simulink model "Proj4_FINAL_INDIVIDUAL"  (R2024b)
settings: Solver=ode15s  StartTime=0.0  StopTime=3600  FixedStep=0.1  MaxStep=1e-2  MinStep=1e-8  RelTol=1e-2  AbsTol=1e-6
values from neighbouring files (symbols this model uses):
  axel_distances = [1.6,1.4]    [Project4_FINAL_INDIVIDUAL_INITIAL.m]
  eta_speed = [0:500:10000]    [Project4_FINAL_INDIVIDUAL_INITIAL.m]
  eta_torque = [0:25:325] * 280/325 * scaleFactor    [Project4_FINAL_INDIVIDUAL_INITIAL.m]
  eta_val = eta_val .* eta_val    [Project4_FINAL_INDIVIDUAL_INITIAL.m]
  g_b = 2.1    [Project4_FINAL_INDIVIDUAL_INITIAL.m]
  gear_ratio = 10    [Project4_FINAL_INDIVIDUAL_INITIAL.m]
  I_w = 1.7    [Project4_FINAL_INDIVIDUAL_INITIAL.m]
  l = 2    [Project4_FINAL_INDIVIDUAL_INITIAL.m]
  lambda_max = 0.1    [Project4_FINAL_INDIVIDUAL_INITIAL.m]
  m = 80    [Project4_FINAL_INDIVIDUAL_INITIAL.m]
  mass_inert = [80,1]    [Project4_FINAL_INDIVIDUAL_INITIAL.m]
  maxtorque = [0, 0, 0, 0, 0, 0,  0,  0,  0,  0,   0,   0,     0 ... (first row only)    [Project4_FINAL_INDIVIDUAL_INITIAL.m]
  mu = 0.8    [Project4_FINAL_INDIVIDUAL_INITIAL.m]
  mu_b = 0.7    [Project4_FINAL_INDIVIDUAL_INITIAL.m]
  N_b_max = 10000    [Project4_FINAL_INDIVIDUAL_INITIAL.m]
  nom_stiff = 50    [Project4_FINAL_INDIVIDUAL_INITIAL.m]
  numParallel = 74    [Project4_FINAL_INDIVIDUAL_INITIAL.m]
  numSeries = 96    [Project4_FINAL_INDIVIDUAL_INITIAL.m]
  OCV = [0, 3.1,3.55,3.68,3.74,3.76,3.78,3.85,3.9,3.95,4.08,4.15]    [Project4_FINAL_INDIVIDUAL_INITIAL.m]
  r_w = 1.4    [Project4_FINAL_INDIVIDUAL_INITIAL.m]
  Rint = 0.1695    [Project4_FINAL_INDIVIDUAL_INITIAL.m]
  rpm = [0,  1000,2000,3000,4000,5000,6000,7000,8000,9000,10000,11000, 12000]    [Project4_FINAL_INDIVIDUAL_INITIAL.m]
  SOC = [0, 0.01,   .1,  .2,  .3,  .4,  .5,  .6, .7,  .8,  .9,   1]    [Project4_FINAL_INDIVIDUAL_INITIAL.m]
  stiffs = [200,180]    [Project4_FINAL_INDIVIDUAL_INITIAL.m]
  v_max = 22    [Project4_FINAL_INDIVIDUAL_INITIAL.m]
  vbus = [250, 350, 500, 600, 700]*scaleFactor    [Project4_FINAL_INDIVIDUAL_INITIAL.m]
  x_center = [x_straightB, x_curveR, x_straightT, x_curveL]    [Project4_FINAL_INDIVIDUAL_INITIAL.m]
  y_center = [y_straightB, y_curveR, y_straightT, y_curveL]    [Project4_FINAL_INDIVIDUAL_INITIAL.m]
libraries: slpidlib x1
settings Model: Creator=davsc  LastModifiedBy=lukep

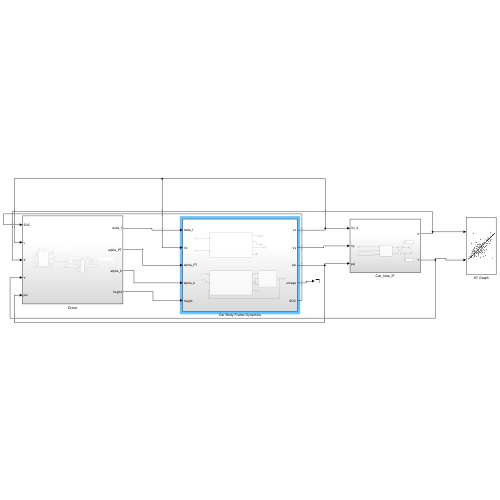
[thumbnail: Simulink's stored preview of the top-level diagram]
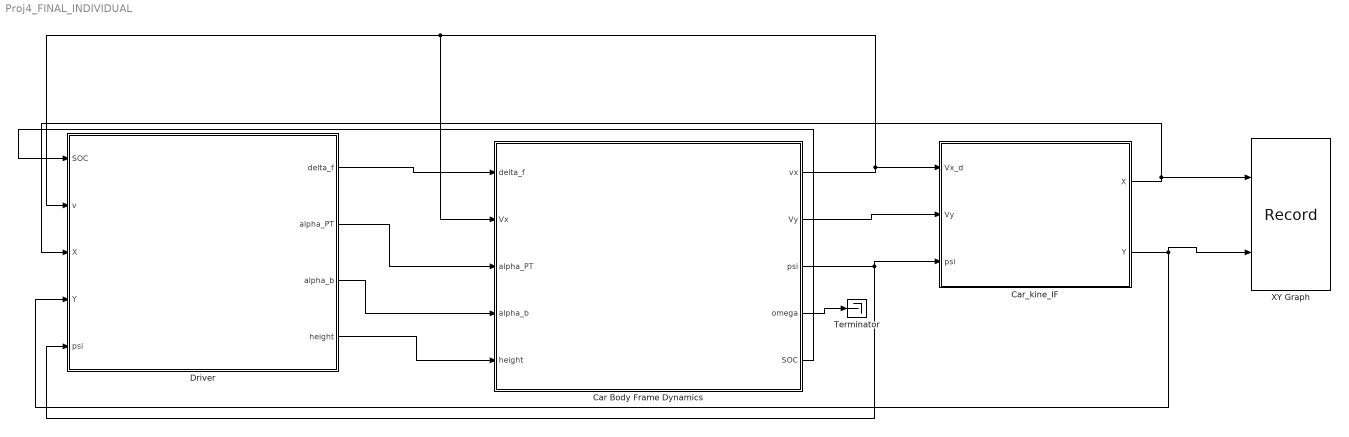
== system Proj4_FINAL_INDIVIDUAL ==
  Car Body Frame Dynamics : Subsystem
  Car_kine_IF : Subsystem
  Driver : Subsystem
  Terminator : Terminator
  XY Graph : Record  FileSettingsInternal="{\"entries\":[{\"content\":{\"excelSettings\":{\"content\":{},\"type\":\"Streamout.ExcelSettings\"}},\"type\":\"Streamout.FileSettingStorage\",\"uuid\":\"\"}],\"packageUris\":[\"http:\\/\\/schema.mathworks.com\\/mf0\\/streamout_blocks\\/R2020a\"],\"version\":\"1.0\"}"  Layout=[1 1]  SignalsInternal="{\"entries\":[{\"content\":{\"signals\":[{\"content\":{\"blockPath\":[],\"dimensions\":[1],\"domain\":\"\",\"lineColor\":\"#edb120\",\"lineWidth\":2,\"port\":1,\"sid\":[\"\"],\"signalID\":1,\"signalName\":\"Car_kine_IF:1\"},\"type\":\"RecordBlkView.Signal\",\"uuid\":\"\"},{\"content\":{\"blockPath\":[],\"dimensions\":[1],\"domain\":\"\",\"lineColor\":\"#7e2f8e\",\"lineWidth\":2,\"port\":2,\"sid\":[\"\"],\"signalID\":2,\"signalName\":\"Car_kine_IF:2\"},\"type\":\"RecordBlkView.Signal\",\"uuid\":\"\"},{\"content\":{\"blockPath\":[],\"dimensions\":[1],\"domain\":\"\",\"lineColor\":\"#77ac30\",\"lineWidth\":2,\"port\":1,\"sid\":[\"\"],\"signalID\":3,\"signalName\":\"MATLAB Function\"},\"type\":\"RecordBlkView.Signal\",\"uuid\":\"\"},{\"content\":{\"blockPath\":[],\"dimensions\":[1],\"domain\":\"\",\"lineColor\":\"#4dbeee\",\"lineWidth\":2,\"port\":1,\"sid\":[\"\"],\"signalID\":4,\"signalName\":\"Integrator\"},\"type\":\"RecordBlkView.Signal\",\"uuid\":\"\"},{\"content\":{\"blockPath\":[],\"dimensions\":[1],\"domain\":\"\",\"lineColor\":\"#a2142f\",\"lineWidth\":2,\"port\":1,\"sid\":[\"\"],\"signalID\":5,\"signalName\":\"Electric Motor Drive:5\"},\"type\":\"RecordBlkView.Signal\",\"uuid\":\"\"},{\"content\":{\"blockPath\":[],\"dimensions\":[1],\"domain\":\"\",\"lineColor\":\"#139fff\",\"lineWidth\":2,\"port\":1,\"sid\":[\"\"],\"signalID\":6,\"signalName\":\"1-D Lookup\\nTable\"},\"type\":\"RecordBlkView.Signal\",\"uuid\":\"\"},{\"content\":{\"blockPath\":[],\"dimensions\":[1],\"domain\":\"\",\"lineColor\":\"#ff6929\",\"lineWidth\":2,\"port\":1,\"sid\":[\"\"],\"signalID\":7,\"signalName\":\"gainn\"},\"type\":\"RecordBlkView.Signal\",\"uuid\":\"\"},{\"content\":{\"blockPath\":[],\"dimensions\":[1],\"domain\":\"\",\"lineColor\":\"#b746ff\",\"lineWidth\":2,\"port\":1,\"sid\":[\"\"],\"signalID\":8,\"signalName\":\"Integrator1\"},\"type\":\"RecordBlkView.Signal\",\"uuid\":\"\"},{\"content\":{\"blockPath\":[],\"dimensions\":[1],\"domain\":\"\",\"lineColor\":\"#64d413\",\"lineWidth\":2,\"port\":1,\"sid\":[\"\"],\"signalID\":9,\"signalName\":\"Motor Efficiency Table\"},\"type\":\"RecordBlkView.Signal\",\"uuid\":\"\"},{\"content\":{\"blockPath\":[],\"dimensions\":[1],\"domain\":\"\",\"lineColor\":\"#ff13a6\",\"lineWidth\":2,\"port\":1,\"sid\":[\"\"],\"signalID\":10,\"signalName\":\"Product1\"},\"type\":\"RecordBlkView.Signal\",\"uuid\":\"\"},{\"content\":{\"blockPath\":[],\"dimensions\":[1],\"domain\":\"\",\"lineColor\":\"#fe330a\",\"lineWidth\":2,\"port\":1,\"sid\":[\"\"],\"signalID\":11,\"signalName\":\"Integrator\"},\"type\":\"RecordBlkView.Signal\",\"uuid\":\"\"},{\"content\":{\"blockPath\":[],\"dimensions\":[1],\"domain\":\"\",\"lineColor\":\"#22b573\",\"lineWidth\":2,\"port\":1,\"sid\":[\"\"],\"signalID\":12,\"signalName\":\"MATLAB Function1:1\"},\"type\":\"RecordBlkView.Signal\",\"uuid\":\"\"},{\"content\":{\"blockPath\":[],\"dimensions\":[1],\"domain\":\"\",\"lineColor\":\"#0072bd\",\"lineWidth\":2,\"port\":1,\"sid\":[\"\"],\"signalID\":13,\"signalName\":\"MATLAB Function1:2\"},\"type\":\"RecordBlkView.Signal\",\"uuid\":\"\"},{\"content\":{\"blockPath\":[],\"dimensions\":[1],\"domain\":\"\",\"lineColor\":\"#d95319\",\"lineWidth\":2,\"port\":1,\"sid\":[\"\"],\"signalID\":14,\"signalName\":\"MATLAB Function2:1\"},\"type\":\"RecordBlkView.Signal\",\"uuid\":\"\"},{\"content\":{\"blockPath\":[],\"dimensions\":[1],\"domain\":\"\",\"lineColor\":\"#edb120\",\"lineWidth\":2,\"port\":1,\"sid\":[\"\"],\"signalID\":15,\"signalName\":\"MATLAB Function2:2\"},\"type\":\"RecordBlkView.Signal\",\"uuid\":\"\"},{\"content\":{\"blockPath\":[],\"dimensions\":[1],\"domain\":\"\",\"lineColor\":\"#7e2f8e\",\"lineWidth\":2,\"port\":1,\"sid\":[\"\"],\"signalID\":16,\"signalName\":\"Integrator2\"},\"type\":\"RecordBlkView.Signal\",\"uuid\":\"\"},{\"content\":{\"blockPath\":[],\"dimensions\":[1],\"domain\":\"\",\"lineColor\":\"#77ac30\",\"lineWidth\":2,\"port\":1,\"sid\":[\"\"],\"signalID\":17,\"signalName\":\"Integrator1\"},\"type\":\"RecordBlkView.Signal\",\"uuid\":\"\"},{\"content\":{\"blockPath\":[],\"dimensions\":[1],\"domain\":\"\",\"lineColor\":\"#4dbeee\",\"lineWidth\":2,\"port\":1,\"sid\":[\"\"],\"signalID\":18,\"signalName\":\"Integrator4\"},\"type\":\"RecordBlkView.Signal\",\"uuid\":\"\"},{\"content\":{\"blockPath\":[],\"dimensions\":[1],\"domain\":\"\",\"lineColor\":\"#a2142f\",\"lineWidth\":2,\"port\":1,\"sid\":[\"\"],\"signalID\":19,\"signalName\":\"Integrator\"},\"type\":\"RecordBlkView.Signal\",\"uuid\":\"\"},{\"content\":{\"blockPath\":[],\"dimensions\":[1],\"domain\":\"\",\"lineColor\":\"#139fff\",\"lineWidth\":2,\"port\":1,\"sid\":[\"\"],\"signalID\":20,\"signalName\":\"Integrator1\"},\"type\":\"RecordBlkView.Signal\",\"uuid\":\"\"},{\"content\":{\"blockPath\":[],\"dimensions\":[1],\"domain\":\"\",\"lineColor\":\"#ff6929\",\"lineWidth\":2,\"port\":1,\"sid\":[\"\"],\"signalID\":21,\"signalName\":\"MATLAB Function:1\"},\"type\":\"RecordBlkView.Signal\",\"uuid\":\"\"},{\"content\":{\"blockPath\":[],\"dimensions\":[1],\"domain\":\"\",\"lineColor\":\"#b746ff\",\"lineWidth\":2,\"port\":1,\"sid\":[\"\"],\"signalID\":22,\"signalName\":\"MATLAB Function:2\"},\"type\":\"RecordBlkView.Signal\",\"uuid\":\"\"}]},\"type\":\"RecordBlkView.InputSignals\",\"uuid\":\"\"}],\"packageUris\":[\"http:\\/\\/schema.mathworks.com\\/mf0\\/streamout_blocks\\/R2020a\"],\"version\":\"1.0\"}"  VisualizationBindings="{\"xyplotplugin\":{\"info\":[{\"series\":[],\"subplotID\":1}]}}"  CompatibilityTag=XY
  wires:
  Driver/2(alpha_PT) -> Car Body Frame Dynamics/3(alpha_PT)
  Driver/3(alpha_b) -> Car Body Frame Dynamics/4(alpha_b)
  Car Body Frame Dynamics/4(omega) -> Terminator/1
  Car Body Frame Dynamics/5(SOC) -> Driver/1(SOC)
  Car Body Frame Dynamics/1(vx) -> Car Body Frame Dynamics/2(Vx), Driver/2(v), Car_kine_IF/1(Vx_d)
  Car Body Frame Dynamics/2(Vy) -> Car_kine_IF/2(Vy)
  Car Body Frame Dynamics/3(psi) -> Car_kine_IF/3(psi), Driver/5(psi)
  Car_kine_IF/1(X) -> Driver/3(X), XY Graph/1
  Car_kine_IF/2(Y) -> XY Graph/2, Driver/4(Y)
  Driver/1(delta_f) -> Car Body Frame Dynamics/1(delta_f)
  Driver/4(height) -> Car Body Frame Dynamics/5(height)

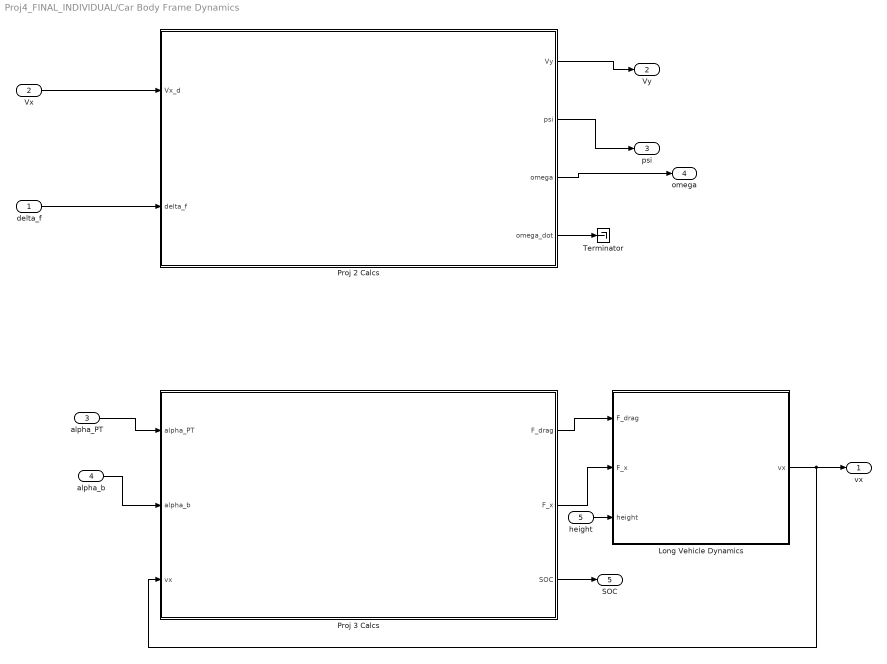
== system Proj4_FINAL_INDIVIDUAL/Car Body Frame Dynamics ==
  delta_f : Inport
  Vx : Inport  Port=2
  alpha_PT : Inport  Port=3
  alpha_b : Inport  Port=4
  height : Inport  Port=5
  Long Vehicle Dynamics : Subsystem
  Proj 2 Calcs : Subsystem
  Proj 3 Calcs : Subsystem
  Terminator : Terminator
  vx : Outport
  Vy : Outport  Port=2
  psi : Outport  Port=3
  omega : Outport  Port=4
  SOC : Outport  Port=5
  wires:
  alpha_PT/1 -> Proj 3 Calcs/1(alpha_PT)
  alpha_b/1 -> Proj 3 Calcs/2(alpha_b)
  Vx/1 -> Proj 2 Calcs/1(Vx_d)
  delta_f/1 -> Proj 2 Calcs/2(delta_f)
  Proj 3 Calcs/2(F_x) -> Long Vehicle Dynamics/2(F_x)
  Proj 3 Calcs/1(F_drag) -> Long Vehicle Dynamics/1(F_drag)
  Proj 3 Calcs/3(SOC) -> SOC/1
  Proj 2 Calcs/1(Vy) -> Vy/1
  Proj 2 Calcs/2(psi) -> psi/1
  Proj 2 Calcs/3(omega) -> omega/1
  Long Vehicle Dynamics/1(vx) -> Proj 3 Calcs/3(vx), vx/1
  Proj 2 Calcs/4(omega_dot) -> Terminator/1
  height/1 -> Long Vehicle Dynamics/3(height)

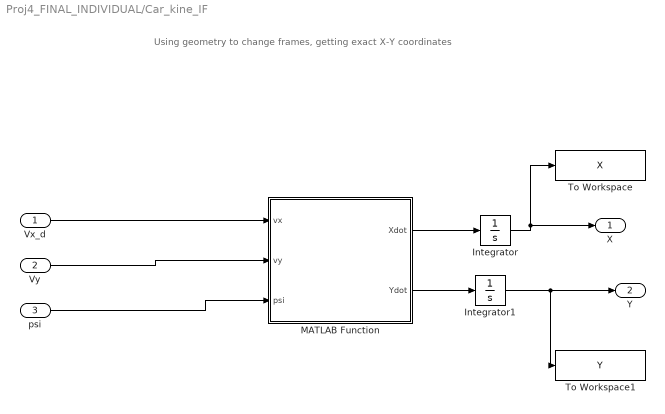
== system Proj4_FINAL_INDIVIDUAL/Car_kine_IF ==
  note: Using geometry to change frames, getting exact X-Y coordinates
  Vx_d : Inport
  Vy : Inport  Port=2
  psi : Inport  Port=3
  Integrator : Integrator
  Integrator1 : Integrator
  MATLAB Function : MATLAB Function  TreatAsAtomicUnit=on
  To Workspace : ToWorkspace  VariableName=X  SaveFormat=Timeseries  SampleTime=0.5
  To Workspace1 : ToWorkspace  VariableName=Y  SaveFormat=Timeseries  SampleTime=0.5
  X : Outport
  Y : Outport  Port=2
  wires:
  Vx_d/1 -> MATLAB Function/1(vx)
  psi/1 -> MATLAB Function/3(psi)
  Vy/1 -> MATLAB Function/2(vy)
  MATLAB Function/1(Xdot) -> Integrator/1
  MATLAB Function/2(Ydot) -> Integrator1/1
  Integrator1/1 -> To Workspace1/1, Y/1
  Integrator/1 -> To Workspace/1, X/1

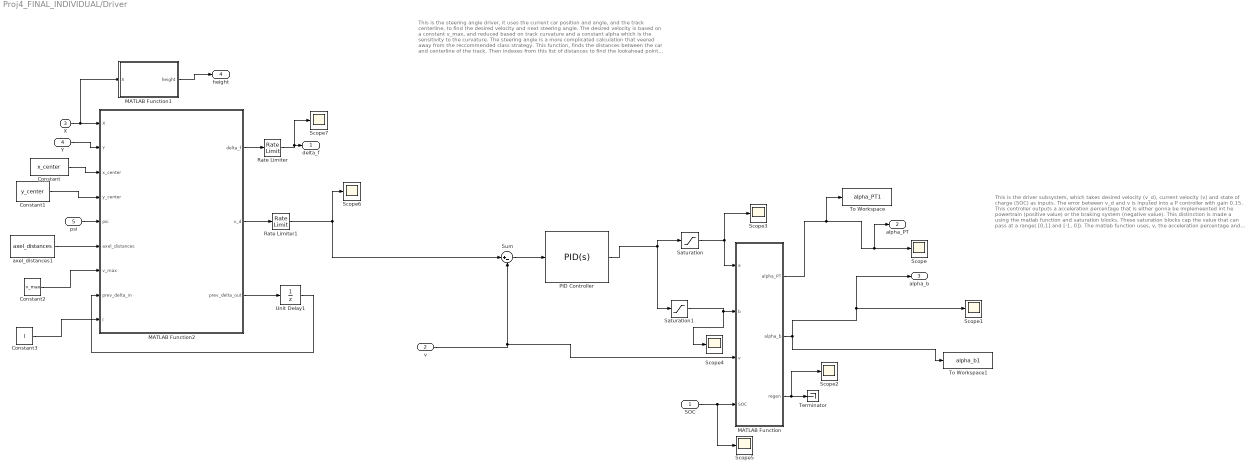
== system Proj4_FINAL_INDIVIDUAL/Driver ==
  note: This is the steering angle driver, it uses the current car position and angle, and the track centerline, to find the desired velocity and next steering angle. The desired velocity is based on a constant v_max, and reduced based on track curvature and a constant alpha which is the sensitivity to the curvature. The steering angle is a more complicated calculation that veered away from the reccommended class strategy. This function, finds the distances between the car and centerline of the track. Then indexes from this list of distances to find the lookahead point on the centerline (distance l). Then steering angle is simply calculated once lookahead point is found (psi_d to error to dleta_f). Where steering angle and desired speed is capped to keep the car on the track as much as possible
  note: This is the driver subsystem, which takes desired velocity (v_d), current velocity (v) and state of charge (SOC) as inputs. The error between v_d and v is inputed into a P controller with gain 0.15. This controller outputs a acceleration percentage that is either gonna be implemeented int he powertrain (positive value) or the braking system (negative value). This distinction is made a using the matlab function and saturation blocks. These saturation blocks cap the value that can pass at a range( [0,1] and [-1, 0]). The matlab function uses, v, the acceleration percentage and SOC, to output the brake or powertrain accerlation and a regeneration factor. The logic of this function accelerates the vehicle based on current speed and current SOC.
  SOC : Inport
  v : Inport  Port=2
  X : Inport  Port=3
  Y : Inport  Port=4
  psi : Inport  Port=5
  Constant : Constant  Value=x_center
  Constant1 : Constant  Value=y_center
  Constant2 : Constant  Value=v_max
  Constant3 : Constant  Value=l
  MATLAB Function : MATLAB Function  TreatAsAtomicUnit=on
  MATLAB Function1 : MATLAB Function  TreatAsAtomicUnit=on
  MATLAB Function2 : MATLAB Function  TreatAsAtomicUnit=on
  PID Controller : slpidlib/PID Controller  Controller=PID  Form=Parallel  TimeDomain=Continuous-time  UseExternalTs=off  SampleTime=-1  IntegratorMethod=Forward Euler  FilterMethod=Forward Euler  ControllerParametersSource=internal  P=0.5  I=0  UseKiTs=off  D=0  UseExternalDerivativeSource=off  N=100  UseFilter=on  TunerSelectOption=Transfer Function Based (PID Tuner App)  InitialConditionSource=internal  InitialConditionForIntegrator=0  InitialConditionForFilter=0  DifferentiatorICPrevScaledInput=0  ExternalReset=none  TrackingMode=off  Kt=1  LimitOutput=off  SatLimitsSource=internal  UpperSaturationLimit=inf  LowerSaturationLimit=-inf  LinearizeAsGain=on  AntiWindupMode=none  Kb=1  LimitIntegrator=off  UpperIntegratorSaturationLimit=inf  LowerIntegratorSaturationLimit=-inf  POutMin=[]  POutMax=[]  IOutMin=[]  IOutMax=[]  DOutMin=[]  DOutMax=[]  NOutMin=[]  NOutMax=[]  SumOutMin=[]  SumOutMax=[]  SaturationOutMin=[]  SaturationOutMax=[]  PParamMin=[]  PParamMax=[]  IParamMin=[]  IParamMax=[]  DParamMin=[]  DParamMax=[]  NParamMin=[]  NParamMax=[]  KbParamMin=[]  KbParamMax=[]  KtParamMin=[]  KtParamMax=[]  KbOutMin=[]  KbOutMax=[]  KtOutMin=[]  KtOutMax=[]  IntegratorOutMin=[]  IntegratorOutMax=[]  FilterOutMin=[]  FilterOutMax=[]  SumI1OutMin=[]  SumI1OutMax=[]  SumI2OutMin=[]  SumI2OutMax=[]  SumI3OutMin=[]  SumI3OutMax=[]  SumI4OutMin=[]  SumI4OutMax=[]  SumDOutMin=[]  SumDOutMax=[]  DifferentiatorOutMin=[]  DifferentiatorOutMax=[]  FilterDiffOutCoefMin=[]  FilterDiffOutCoefMax=[]  ReciprocalOutMin=[]  ReciprocalOutMax=[]  SumDenOutMin=[]  SumDenOutMax=[]  SumNumOutMin=[]  SumNumOutMax=[]  DivideOutMin=[]  DivideOutMax=[]  UdiffTsProdOutMin=[]  UdiffTsProdOutMax=[]  NTsProdOutMin=[]  NTsProdOutMax=[]  UintegralTsProdOutMin=[]  UintegralTsProdOutMax=[]  UngainTsProdOutMin=[]  UngainTsProdOutMax=[]  ClampingZeroOutDataTypeStr=Inherit: Inherit via back propagation  ClampingZeroOutMin=[]  ClampingZeroOutMax=[]  FilterDenConstantOutDataTypeStr=Inherit: Inherit via back propagation  FilterDenConstantOutMin=[]  FilterDenConstantOutMax=[]  PCopyOutDataTypeStr=Inherit: Inherit via back propagation  PCopyOutMin=[]  PCopyOutMax=[]  NCopyOutDataTypeStr=Inherit: Inherit via back propagation  NCopyOutMin=[]  NCopyOutMax=[]  IntegratorContinuousStateAttributes=''  IntegratorStateMustResolveToSignalObject=off  IntegratorRTWStateStorageClass=Auto  FilterContinuousStateAttributes=''  FilterStateMustResolveToSignalObject=off  FilterRTWStateStorageClass=Auto  ParallelPVariant=InternalParameters  IdealPVariant=Disabled  IVariant=InternalParameters  DVariant=InternalParameters  IntegratorVariant=Continuous  SatVariant=Disabled  AWVariant=Passthrough  PCopyVariant=Disabled  TRVariant=Disabled  FdbkBlocksVariant=Forward  IdealPFdbkVariant=Disabled  SatFdbkVariant=Disabled  DerivativeFilterVariant=ContFilter  NVariant=InternalParameters  NCopyVariant=Disabled  FilterICVariant=InternalICsFilter  IntegratorICVariant=InternalICs  ExternalResetVariant=Disabled  TRSumVariant=Passthrough  SumFdbkVariant=Disabled  SumVariant=Sum_PID  TsampFilterVariant=InternalTs  TsampNgainVariant=Passthrough  TsampIntegralVariant=Disabled_SignalSpec  ExternalSaturationOutDataTypeStr=Inherit: Same as second input  DerivativeSourceVariant=ErrorSignal  PreIntVariant=InternalPreInt
  Rate Limiter : RateLimiter  SampleTimeMode=inherited
  Rate Limiter1 : RateLimiter  SampleTimeMode=inherited
  Saturation : Saturate  UpperLimit=1  LowerLimit=0
  Saturation1 : Saturate  UpperLimit=0  LowerLimit=-1
  Scope{,1..7} (8 alike) : Scope
  Sum : Sum  Inputs=|+-
  Terminator : Terminator
  To Workspace : ToWorkspace  VariableName=alpha_PT1  SaveFormat=Timeseries  SampleTime=-1
  To Workspace1 : ToWorkspace  VariableName=alpha_b1  SaveFormat=Timeseries  SampleTime=-1
  Unit Delay1 : UnitDelay  SampleTime=-1  HasFrameUpgradeWarning=on
  axel_distances1 : Constant  Value=axel_distances
  delta_f : Outport
  alpha_PT : Outport  Port=2
  alpha_b : Outport  Port=3
  height : Outport  Port=4
  wires:
  Sum/1 -> PID Controller/1
  PID Controller/1 -> Saturation/1, Saturation1/1
  MATLAB Function2/2(v_d) -> Rate Limiter1/1
  MATLAB Function/2(alpha_b) -> alpha_b/1, Scope1/1, To Workspace1/1
  MATLAB Function/3(regen) -> Scope2/1, Terminator/1
  Saturation1/1 -> Scope4/1, MATLAB Function/2(b)
  SOC/1 -> Scope5/1, MATLAB Function/4(SOC)
  Saturation/1 -> MATLAB Function/1(a), Scope3/1
  v/1 -> MATLAB Function/3(v), Sum/2
  MATLAB Function/1(alpha_PT) -> To Workspace/1, Scope/1, alpha_PT/1
  axel_distances1/1 -> MATLAB Function2/6(axel_distances)
  MATLAB Function2/3(prev_delta_out) -> Unit Delay1/1
  Constant3/1 -> MATLAB Function2/9(l)
  Constant2/1 -> MATLAB Function2/7(v_max)
  Constant1/1 -> MATLAB Function2/4(y_center)
  X/1 -> MATLAB Function1/1(X), MATLAB Function2/1(X)
  Y/1 -> MATLAB Function2/2(Y)
  Constant/1 -> MATLAB Function2/3(x_center)
  psi/1 -> MATLAB Function2/5(psi)
  Unit Delay1/1 -> MATLAB Function2/8(prev_delta_in)
  MATLAB Function2/1(delta_f) -> Rate Limiter/1
  Rate Limiter/1 -> Scope7/1, delta_f/1
  Rate Limiter1/1 -> Scope6/1, Sum/1
  MATLAB Function1/1(height) -> height/1

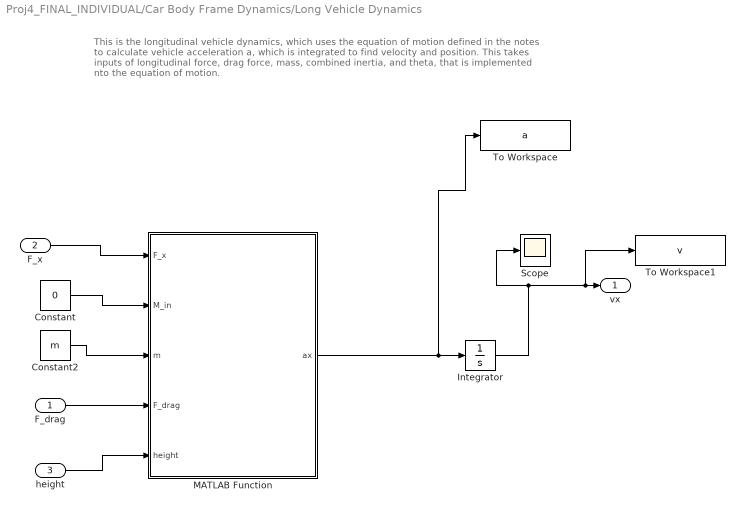
== system Proj4_FINAL_INDIVIDUAL/Car Body Frame Dynamics/Long Vehicle Dynamics ==
  note: This is the longitudinal vehicle dynamics, which uses the equation of motion defined in the notes to calculate vehicle acceleration a, which is integrated to find velocity and position. This takes inputs of longitudinal force, drag force, mass, combined inertia, and theta, that is implemented nto the equation of motion.
  F_drag : Inport
  F_x : Inport  Port=2
  height : Inport  Port=3
  Constant : Constant  Value=0
  Constant2 : Constant  Value=m
  Integrator : Integrator  InitialCondition=0.1
  MATLAB Function : MATLAB Function  TreatAsAtomicUnit=on
  Scope : Scope
  To Workspace : ToWorkspace  VariableName=a  SaveFormat=Timeseries  SampleTime=-1
  To Workspace1 : ToWorkspace  VariableName=v  SaveFormat=Timeseries  SampleTime=-1
  vx : Outport
  wires:
  F_drag/1 -> MATLAB Function/4(F_drag)
  F_x/1 -> MATLAB Function/1(F_x)
  Constant/1 -> MATLAB Function/2(M_in)
  Constant2/1 -> MATLAB Function/3(m)
  MATLAB Function/1(ax) -> To Workspace/1, Integrator/1
  Integrator/1 -> Scope/1, To Workspace1/1, vx/1
  height/1 -> MATLAB Function/5(height)

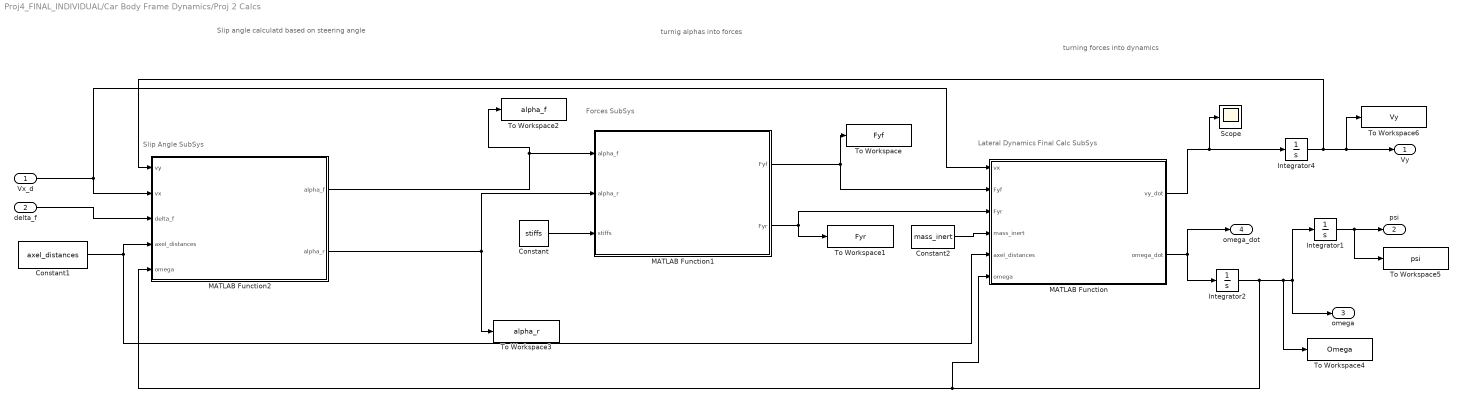
== system Proj4_FINAL_INDIVIDUAL/Car Body Frame Dynamics/Proj 2 Calcs ==
  note: turning forces into dynamics
  note: turnig alphas into forces
  note: Slip angle calculatd based on steering angle
  note: Forces SubSys
  note: Slip Angle SubSys
  note: Lateral Dynamics Final Calc SubSys
  Vx_d : Inport
  delta_f : Inport  Port=2
  Constant : Constant  Value=stiffs
  Constant1 : Constant  Value=axel_distances
  Constant2 : Constant  Value=mass_inert
  Integrator1 : Integrator
  Integrator2 : Integrator
  Integrator4 : Integrator
  MATLAB Function : MATLAB Function  TreatAsAtomicUnit=on
  MATLAB Function1 : MATLAB Function  TreatAsAtomicUnit=on
  MATLAB Function2 : MATLAB Function  TreatAsAtomicUnit=on
  Scope : Scope
  To Workspace : ToWorkspace  VariableName=Fyf  SaveFormat=Timeseries  SampleTime=-1
  To Workspace1 : ToWorkspace  VariableName=Fyr  SaveFormat=Timeseries  SampleTime=-1
  To Workspace2 : ToWorkspace  VariableName=alpha_f  SaveFormat=Timeseries  SampleTime=-1
  To Workspace3 : ToWorkspace  VariableName=alpha_r  SaveFormat=Timeseries  SampleTime=-1
  To Workspace4 : ToWorkspace  VariableName=Omega  SaveFormat=Timeseries  SampleTime=-1
  To Workspace5 : ToWorkspace  VariableName=psi  SaveFormat=Timeseries  SampleTime=-1
  To Workspace6 : ToWorkspace  VariableName=Vy  SaveFormat=Timeseries  SampleTime=-1
  Vy : Outport
  psi : Outport  Port=2
  omega : Outport  Port=3
  omega_dot : Outport  Port=4
  wires:
  Vx_d/1 -> MATLAB Function/1(vx), MATLAB Function2/2(vx)
  Integrator4/1 -> MATLAB Function2/1(vy), To Workspace6/1, Vy/1
  MATLAB Function/1(vy_dot) -> Scope/1, Integrator4/1
  Constant1/1 -> MATLAB Function/5(axel_distances), MATLAB Function2/4(axel_distances)
  Integrator1/1 -> To Workspace5/1, psi/1
  MATLAB Function2/2(alpha_r) -> MATLAB Function1/2(alpha_r), To Workspace3/1
  MATLAB Function1/1(Fyf) -> MATLAB Function/2(Fyf), To Workspace/1
  delta_f/1 -> MATLAB Function2/3(delta_f)
  MATLAB Function/2(omega_dot) -> omega_dot/1, Integrator2/1
  Integrator2/1 -> MATLAB Function2/5(omega), MATLAB Function/6(omega), To Workspace4/1, Integrator1/1, omega/1
  Constant2/1 -> MATLAB Function/4(mass_inert)
  MATLAB Function2/1(alpha_f) -> To Workspace2/1, MATLAB Function1/1(alpha_f)
  Constant/1 -> MATLAB Function1/3(stiffs)
  MATLAB Function1/2(Fyr) -> MATLAB Function/3(Fyr), To Workspace1/1

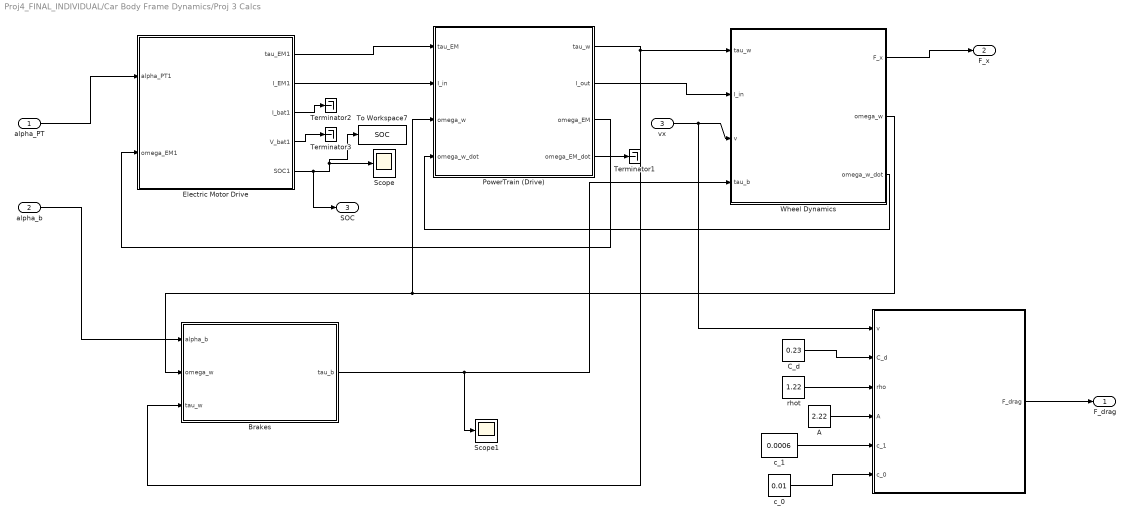
== system Proj4_FINAL_INDIVIDUAL/Car Body Frame Dynamics/Proj 3 Calcs ==
  alpha_PT : Inport
  alpha_b : Inport  Port=2
  vx : Inport  Port=3
  " " : Subsystem
  A : Constant  Value=2.22
  Brakes : Subsystem
  C_d : Constant  Value=0.23
  Electric Motor Drive : Subsystem
  PowerTrain (Drive) : Subsystem
  Scope : Scope
  Scope1 : Scope
  Terminator1 : Terminator
  Terminator2 : Terminator
  Terminator3 : Terminator
  To Workspace7 : ToWorkspace  VariableName=SOC  SaveFormat=Timeseries  SampleTime=-1
  Wheel Dynamics : Subsystem
  c_0 : Constant  Value=0.01
  c_1 : Constant  Value=0.0006
  rhot : Constant  Value=1.22
  F_drag : Outport
  F_x : Outport  Port=2
  SOC : Outport  Port=3
  wires:
  Electric Motor Drive/5(SOC1) -> SOC/1, To Workspace7/1, Scope/1
  A/1 -> " "/4(A)
  Electric Motor Drive/4(V_bat1) -> Terminator3/1
  c_0/1 -> " "/6(c_0)
  rhot/1 -> " "/3(rho)
  Wheel Dynamics/2(omega_w) -> PowerTrain (Drive)/3(omega_w), Brakes/2(omega_w)
  PowerTrain (Drive)/2(I_out) -> Wheel Dynamics/2(I_in)
  Brakes/1(tau_b) -> Scope1/1, Wheel Dynamics/4(tau_b)
  PowerTrain (Drive)/4(omega_EM_dot) -> Terminator1/1
  PowerTrain (Drive)/3(omega_EM) -> Electric Motor Drive/2(omega_EM1)
  Wheel Dynamics/3(omega_w_dot) -> PowerTrain (Drive)/4(omega_w_dot)
  alpha_b/1 -> Brakes/1(alpha_b)
  c_1/1 -> " "/5(c_1)
  PowerTrain (Drive)/1(tau_w) -> Brakes/3(tau_w), Wheel Dynamics/1(tau_w)
  C_d/1 -> " "/2(C_d)
  alpha_PT/1 -> Electric Motor Drive/1(alpha_PT1)
  Electric Motor Drive/1(tau_EM1) -> PowerTrain (Drive)/1(tau_EM)
  Electric Motor Drive/2(I_EM1) -> PowerTrain (Drive)/2(I_in)
  " "/1(F_drag) -> F_drag/1
  Wheel Dynamics/1(F_x) -> F_x/1
  vx/1 -> Wheel Dynamics/3(v), " "/1(v)
  Electric Motor Drive/3(I_bat1) -> Terminator2/1

== system Proj4_FINAL_INDIVIDUAL/Car Body Frame Dynamics/Proj 3 Calcs/  ==
  note: Drag force Subsystem, using constants and current velocity. Implemented in matlab function using given formula in notes.
  v : Inport
  C_d : Inport  Port=2
  rho : Inport  Port=3
  A : Inport  Port=4
  c_1 : Inport  Port=5
  c_0 : Inport  Port=6
  Drag_force : MATLAB Function  TreatAsAtomicUnit=on
  F_drag : Outport
  wires:
  Drag_force/1(F_drag) -> F_drag/1
  C_d/1 -> Drag_force/4(C_d)
  A/1 -> Drag_force/3(A)
  rho/1 -> Drag_force/2(rho)
  v/1 -> Drag_force/1(v)
  c_0/1 -> Drag_force/6(c_0)
  c_1/1 -> Drag_force/5(c_1)

== system Proj4_FINAL_INDIVIDUAL/Car Body Frame Dynamics/Proj 3 Calcs/Brakes ==
  note: This is the brakes subsystem. This takes brake percentage, wheel angular speed (omega_w), and defined constants: max brake force (N_b_max), brake friction (mu_b), and geometric design factor (g_b), and outputs brake torque (tau_b). This is implemented using a given formula in the notes.
  alpha_b : Inport
  omega_w : Inport  Port=2
  tau_w : Inport  Port=3
  Constant : Constant  Value=N_b_max
  Constant1 : Constant  Value=g_b
  Constant2 : Constant  Value=mu_b
  MATLAB Function : MATLAB Function  TreatAsAtomicUnit=on
  tau_b : Outport
  wires:
  Constant2/1 -> MATLAB Function/4(mu_b)
  Constant1/1 -> MATLAB Function/3(g_b)
  Constant/1 -> MATLAB Function/2(N_b_max)
  alpha_b/1 -> MATLAB Function/1(alpha_b)
  omega_w/1 -> MATLAB Function/5(omega_w)
  MATLAB Function/1(tau_b) -> tau_b/1
  tau_w/1 -> MATLAB Function/6(tau_w)

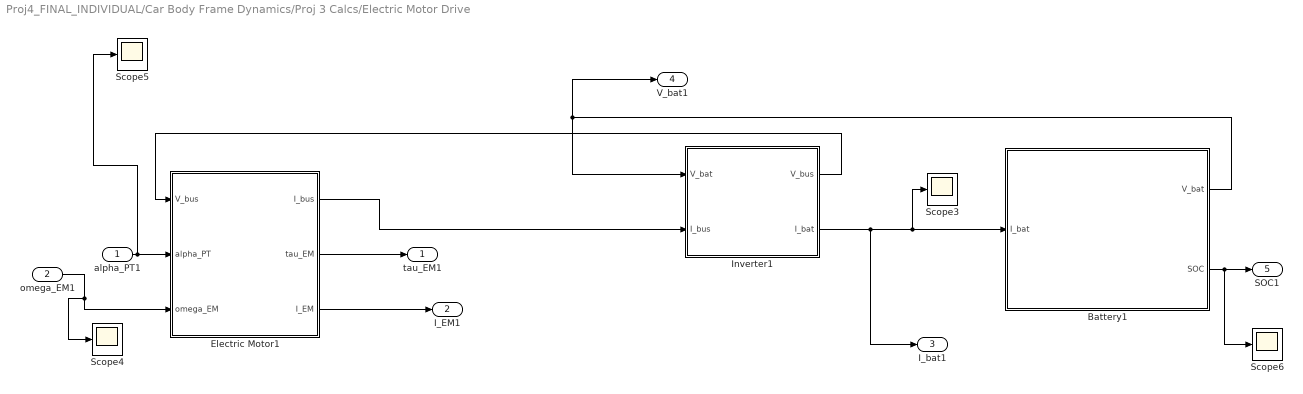
== system Proj4_FINAL_INDIVIDUAL/Car Body Frame Dynamics/Proj 3 Calcs/Electric Motor Drive ==
  alpha_PT1 : Inport
  omega_EM1 : Inport  Port=2
  Battery1 : Subsystem
  Electric Motor1 : Subsystem
  Inverter1 : Subsystem
  Scope{3..6} (4 alike) : Scope
  tau_EM1 : Outport
  I_EM1 : Outport  Port=2
  I_bat1 : Outport  Port=3
  V_bat1 : Outport  Port=4
  SOC1 : Outport  Port=5
  wires:
  Battery1/2(SOC) -> Scope6/1, SOC1/1
  alpha_PT1/1 -> Scope5/1, Electric Motor1/2(alpha_PT)
  Inverter1/1(V_bus) -> Electric Motor1/1(V_bus)
  Battery1/1(V_bat) -> Inverter1/1(V_bat), V_bat1/1
  Electric Motor1/1(I_bus) -> Inverter1/2(I_bus)
  Inverter1/2(I_bat) -> Scope3/1, Battery1/1(I_bat), I_bat1/1
  omega_EM1/1 -> Scope4/1, Electric Motor1/3(omega_EM)
  Electric Motor1/3(I_EM) -> I_EM1/1
  Electric Motor1/2(tau_EM) -> tau_EM1/1

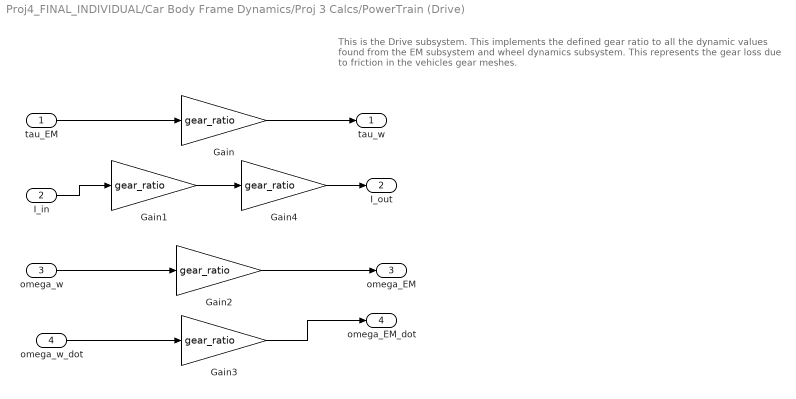
== system Proj4_FINAL_INDIVIDUAL/Car Body Frame Dynamics/Proj 3 Calcs/PowerTrain (Drive) ==
  note: This is the Drive subsystem. This implements the defined gear ratio to all the dynamic values found from the EM subsystem and wheel dynamics subsystem. This represents the gear loss due to friction in the vehicles gear meshes.
  tau_EM : Inport
  I_in : Inport  Port=2
  omega_w : Inport  Port=3
  omega_w_dot : Inport  Port=4
  Gain{,1..4} (5 alike) : Gain  Gain=gear_ratio
  tau_w : Outport
  I_out : Outport  Port=2
  omega_EM : Outport  Port=3
  omega_EM_dot : Outport  Port=4
  wires:
  Gain/1 -> tau_w/1
  tau_EM/1 -> Gain/1
  I_in/1 -> Gain1/1
  omega_w/1 -> Gain2/1
  Gain2/1 -> omega_EM/1
  Gain3/1 -> omega_EM_dot/1
  omega_w_dot/1 -> Gain3/1
  Gain1/1 -> Gain4/1
  Gain4/1 -> I_out/1

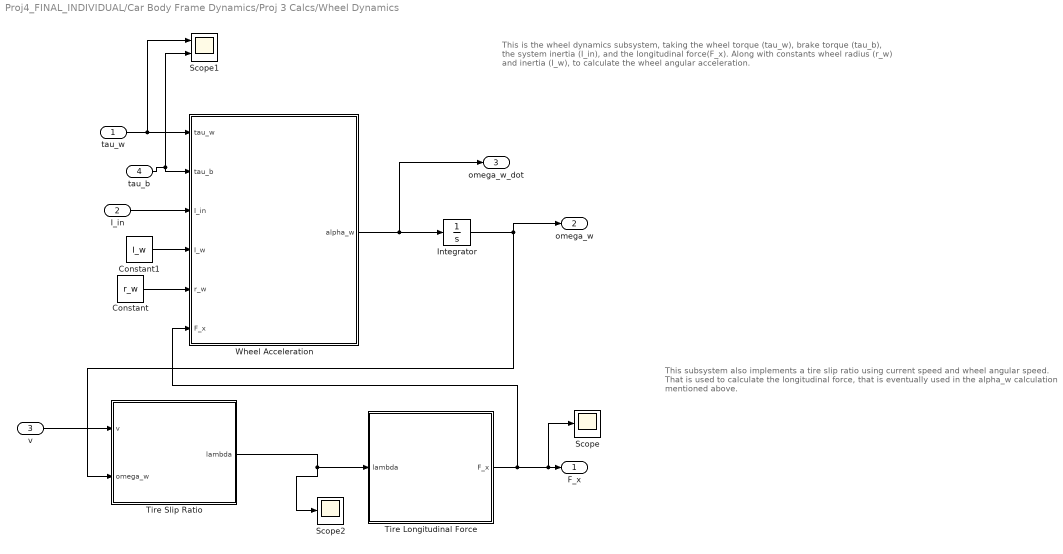
== system Proj4_FINAL_INDIVIDUAL/Car Body Frame Dynamics/Proj 3 Calcs/Wheel Dynamics ==
  note: This is the wheel dynamics subsystem, taking the wheel torque (tau_w), brake torque (tau_b), the system inertia (I_in), and the longitudinal force(F_x). Along with constants wheel radius (r_w) and inertia (I_w), to calculate the wheel angular acceleration.
  note: This subsystem also implements a tire slip ratio using current speed and wheel angular speed. That is used to calculate the longitudinal force, that is eventually used in the alpha_w calculation mentioned above.
  tau_w : Inport
  I_in : Inport  Port=2
  v : Inport  Port=3
  tau_b : Inport  Port=4
  Constant : Constant  Value=r_w
  Constant1 : Constant  Value=I_w
  Integrator : Integrator
  Scope : Scope
  Scope1 : Scope  NumInputPorts=2
  Scope2 : Scope
  Tire Longitudinal Force : Subsystem
  Tire Slip Ratio : Subsystem
  Wheel Acceleration : MATLAB Function  TreatAsAtomicUnit=on
  F_x : Outport
  omega_w : Outport  Port=2
  omega_w_dot : Outport  Port=3
  wires:
  Tire Slip Ratio/1(lambda) -> Scope2/1, Tire Longitudinal Force/1(lambda)
  v/1 -> Tire Slip Ratio/1(v)
  Tire Longitudinal Force/1(F_x) -> Wheel Acceleration/6(F_x), Scope/1, F_x/1
  Constant/1 -> Wheel Acceleration/5(r_w)
  I_in/1 -> Wheel Acceleration/3(I_in)
  Constant1/1 -> Wheel Acceleration/4(I_w)
  tau_w/1 -> Scope1/1, Wheel Acceleration/1(tau_w)
  tau_b/1 -> Scope1/2, Wheel Acceleration/2(tau_b)
  Integrator/1 -> Tire Slip Ratio/2(omega_w), omega_w/1
  Wheel Acceleration/1(alpha_w) -> omega_w_dot/1, Integrator/1

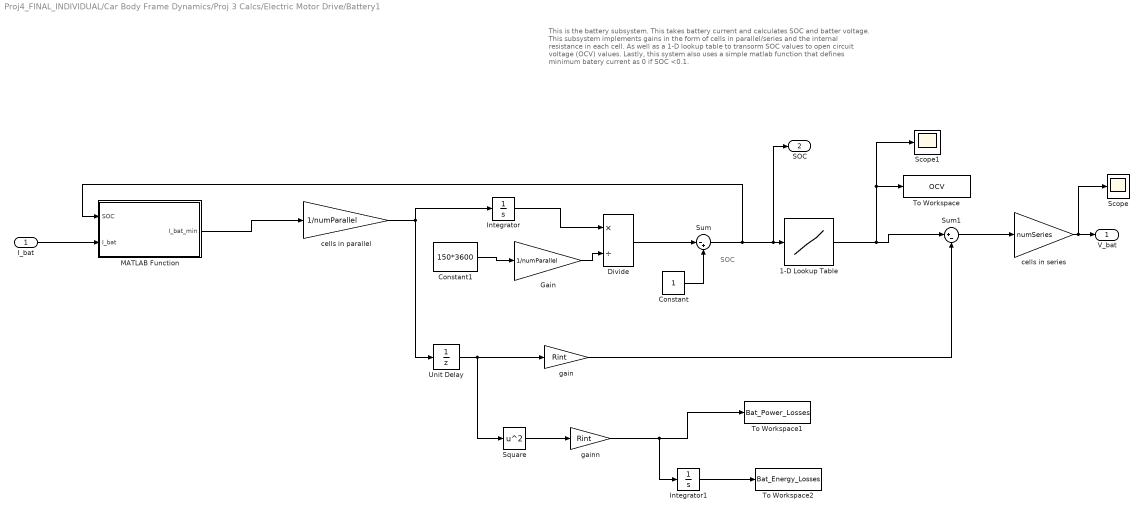
== system Proj4_FINAL_INDIVIDUAL/Car Body Frame Dynamics/Proj 3 Calcs/Electric Motor Drive/Battery1 ==
  note: This is the battery subsystem. This takes battery current and calculates SOC and batter voltage. This subsystem implements gains in the form of cells in parallel/series and the internal resistance in each cell. As well as a 1-D lookup table to transorm SOC values to open circuit voltage (OCV) values. Lastly, this system also uses a simple matlab function that defines minimum batery current as 0 if SOC <0.1.
  note: SOC
  I_bat : Inport
  1-D Lookup Table : Lookup_n-D  NumberOfTableDimensions=1  BreakpointsForDimension1=SOC  Table=OCV  InternalRulePriority=Speed  RndMeth=Simplest
  Constant : Constant
  Constant1 : Constant  Value=150*3600
  Divide : Product  Inputs=*/
  Gain : Gain  Gain=1/numParallel
  Integrator : Integrator
  Integrator1 : Integrator
  MATLAB Function : MATLAB Function  TreatAsAtomicUnit=on
  Scope : Scope
  Scope1 : Scope
  Square : Math  Operator=square
  Sum : Sum  Inputs=|-+
  Sum1 : Sum  Inputs=|+-
  To Workspace : ToWorkspace  VariableName=OCV  SaveFormat=Timeseries  SampleTime=-1
  To Workspace1 : ToWorkspace  VariableName=Bat_Power_Losses  SaveFormat=Timeseries  SampleTime=-1
  To Workspace2 : ToWorkspace  VariableName=Bat_Energy_Losses  SaveFormat=Timeseries  SampleTime=-1
  Unit Delay : UnitDelay  SampleTime=-1  HasFrameUpgradeWarning=on
  cells in parallel : Gain  Gain=1/numParallel
  cells in series : Gain  Gain=numSeries
  gain : Gain  Gain=Rint
  gainn : Gain  Gain=Rint
  V_bat : Outport
  SOC : Outport  Port=2
  wires:
  cells in parallel/1 -> Unit Delay/1, Integrator/1
  MATLAB Function/1(I_bat_min) -> cells in parallel/1
  Integrator/1 -> Divide/1
  Gain/1 -> Divide/2
  Constant1/1 -> Gain/1
  Divide/1 -> Sum/1
  Constant/1 -> Sum/2
  Unit Delay/1 -> Square/1, gain/1
  Square/1 -> gainn/1
  I_bat/1 -> MATLAB Function/2(I_bat)
  Sum/1 -> MATLAB Function/1(SOC), SOC/1, 1-D Lookup Table/1
  gain/1 -> Sum1/2
  1-D Lookup Table/1 -> Scope1/1, To Workspace/1, Sum1/1
  cells in series/1 -> Scope/1, V_bat/1
  Sum1/1 -> cells in series/1
  Integrator1/1 -> To Workspace2/1
  gainn/1 -> To Workspace1/1, Integrator1/1

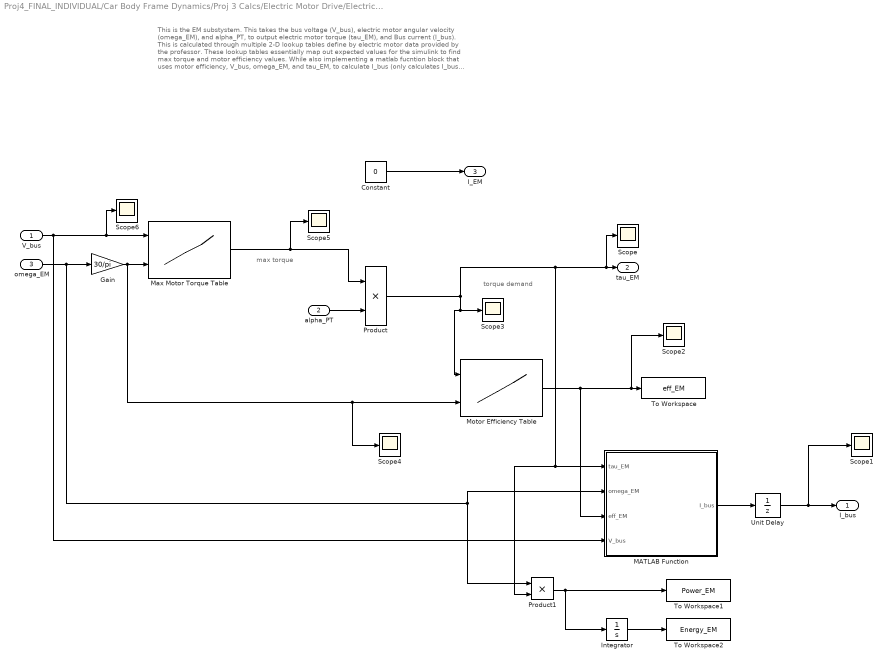
== system Proj4_FINAL_INDIVIDUAL/Car Body Frame Dynamics/Proj 3 Calcs/Electric Motor Drive/Electric Motor1 ==
  note: This is the EM substystem. This takes the bus voltage (V_bus), electric motor angular velocity (omega_EM), and alpha_PT, to output electric motor torque (tau_EM), and Bus current (I_bus). This is calculated through multiple 2-D lookup tables define by electric motor data provided by the professor. These lookup tables essentially map out expected values for the simulink to find max torque and motor efficiency values. While also implementing a matlab fucntion block that uses motor efficiency, V_bus, omega_EM, and tau_EM, to calculate I_bus (only calculates I_bus when V_bus is greater than 1).
  note: torque demand
  note: max torque
  V_bus : Inport
  alpha_PT : Inport  Port=2
  omega_EM : Inport  Port=3
  Constant : Constant  Value=0
  Gain : Gain  Gain=30/pi
  Integrator : Integrator
  MATLAB Function : MATLAB Function  TreatAsAtomicUnit=on
  Max Motor Torque Table : Lookup_n-D  BreakpointsForDimension1=vbus  BreakpointsForDimension2=rpm  Table=maxtorque  InternalRulePriority=Speed  RndMeth=Simplest
      settings: InputPortMap=u0,u1
  Motor Efficiency Table : Lookup_n-D  BreakpointsForDimension1=eta_torque  BreakpointsForDimension2=eta_speed  Table=eta_val  InternalRulePriority=Speed  RndMeth=Simplest
      settings: InputPortMap=u0,u1
  Product : Product
  Product1 : Product
  Scope{,1..6} (7 alike) : Scope
  To Workspace : ToWorkspace  VariableName=eff_EM  SaveFormat=Timeseries  SampleTime=-1
  To Workspace1 : ToWorkspace  VariableName=Power_EM  SaveFormat=Timeseries  SampleTime=-1
  To Workspace2 : ToWorkspace  VariableName=Energy_EM  SaveFormat=Timeseries  SampleTime=-1
  Unit Delay : UnitDelay  SampleTime=-1  HasFrameUpgradeWarning=on
  I_bus : Outport
  tau_EM : Outport  Port=2
  I_EM : Outport  Port=3
  wires:
  Gain/1 -> Scope4/1, Motor Efficiency Table/2, Max Motor Torque Table/2
  omega_EM/1 -> Product1/1, MATLAB Function/2(omega_EM), Gain/1
  V_bus/1 -> Scope6/1, Max Motor Torque Table/1, MATLAB Function/4(V_bus)
  Constant/1 -> I_EM/1
  alpha_PT/1 -> Product/2
  Max Motor Torque Table/1 -> Product/1, Scope5/1
  Motor Efficiency Table/1 -> MATLAB Function/3(eff_EM), Scope2/1, To Workspace/1
  MATLAB Function/1(I_bus) -> Unit Delay/1
  Integrator/1 -> To Workspace2/1
  Product1/1 -> Integrator/1, To Workspace1/1
  Product/1 -> Product1/2, MATLAB Function/1(tau_EM), Scope/1, tau_EM/1, Motor Efficiency Table/1, Scope3/1
  Unit Delay/1 -> I_bus/1, Scope1/1

== system Proj4_FINAL_INDIVIDUAL/Car Body Frame Dynamics/Proj 3 Calcs/Electric Motor Drive/Inverter1 ==
  note: This is the inverter subsystem. This transfers battery to bus electricity values, using a inverter efficiency constant
  V_bat : Inport
  I_bus : Inport  Port=2
  MATLAB Function : MATLAB Function  TreatAsAtomicUnit=on
  Scope{,1..3} (4 alike) : Scope
  eff_inverter : Constant  Value=0.95
  V_bus : Outport
  I_bat : Outport  Port=2
  wires:
  MATLAB Function/1(V_bus) -> Scope1/1, V_bus/1
  MATLAB Function/2(I_bat) -> Scope/1, I_bat/1
  I_bus/1 -> Scope3/1, MATLAB Function/3(I_bus)
  V_bat/1 -> Scope2/1, MATLAB Function/1(V_bat)
  eff_inverter/1 -> MATLAB Function/2(eff_I)

== system Proj4_FINAL_INDIVIDUAL/Car Body Frame Dynamics/Proj 3 Calcs/Wheel Dynamics/Tire Longitudinal Force ==
  lambda : Inport
  Constant : Constant  Value=lambda_max
  Constant1 : Constant  Value=nom_stiff
  Constant2 : Constant  Value=mu
  Constant3 : Constant  Value=m
  MATLAB Function : MATLAB Function  TreatAsAtomicUnit=on
  F_x : Outport
  wires:
  lambda/1 -> MATLAB Function/1(lambda)
  MATLAB Function/1(F_x) -> F_x/1
  Constant/1 -> MATLAB Function/2(lambda_max)
  Constant1/1 -> MATLAB Function/3(nom_stiff)
  Constant2/1 -> MATLAB Function/4(mu)
  Constant3/1 -> MATLAB Function/5(m)

== system Proj4_FINAL_INDIVIDUAL/Car Body Frame Dynamics/Proj 3 Calcs/Wheel Dynamics/Tire Slip Ratio ==
  v : Inport
  omega_w : Inport  Port=2
  Constant : Constant  Value=r_w
  MATLAB Function : MATLAB Function  TreatAsAtomicUnit=on
  lambda : Outport
  wires:
  v/1 -> MATLAB Function/1(v)
  omega_w/1 -> MATLAB Function/2(omega_w)
  Constant/1 -> MATLAB Function/3(r_w)
  MATLAB Function/1(lambda) -> lambda/1

== matlab function Proj4_FINAL_INDIVIDUAL/Car_kine_IF/MATLAB Function ==
  data: vx input; vy input; psi input; Xdot output; Ydot output
function [Xdot, Ydot] = fcn(vx,vy,psi)
    temp = TF(psi)*[vx;vy];
    Xdot = temp(1);
    Ydot = temp(2);

end

function y = TF(psi)
    
    y = [cos(psi), -sin(psi); sin(psi), cos(psi)];

end

== matlab function Proj4_FINAL_INDIVIDUAL/Car Body Frame Dynamics/Proj 3 Calcs/Wheel Dynamics/Tire Longitudinal Force/MATLAB Function ==
  data: lambda input; F_x output; lambda_max input; nom_stiff input; mu input; m input
function F_x = fcn(lambda, lambda_max, nom_stiff, mu, m)

    N = m*9.81/4;

    C_lam = nom_stiff*mu*N;

    if lambda >= 0
        F_x = C_lam*min(lambda_max,lambda);
    else
        F_x =C_lam*max(-lambda_max,lambda);
    end
end

== matlab function Proj4_FINAL_INDIVIDUAL/Car Body Frame Dynamics/Proj 3 Calcs/Wheel Dynamics/Tire Slip Ratio/MATLAB Function ==
  data: v input; lambda output; omega_w input; r_w input
function lambda = fcn(v, omega_w, r_w)

epsilon = 0.0001;

if (r_w*omega_w >= v - epsilon)

    lambda = (r_w*omega_w - v)/(abs(r_w*omega_w)+epsilon);

else

    lambda = (r_w*omega_w - v)/(abs(v)+epsilon);

end

== matlab function Proj4_FINAL_INDIVIDUAL/Car Body Frame Dynamics/Proj 3 Calcs/Wheel Dynamics/Wheel Acceleration ==
  data: tau_w input; alpha_w output; tau_b input; I_in input; I_w input; r_w input; F_x input
function alpha_w = fcn(tau_w, tau_b, I_in, I_w, r_w, F_x)

alpha_w = (tau_w - tau_b - F_x*r_w)/(I_w+I_in);

== matlab function Proj4_FINAL_INDIVIDUAL/Driver/MATLAB Function ==
  data: a input; b input; alpha_PT output; alpha_b output; regen output; v input; SOC input
function [alpha_PT, alpha_b, regen] = fcn(a,b, v, SOC)
    
    speed1 = 5*1600/3600;
    speed2 = 25*1600/3600;
    dspeed = speed2-speed1;

    absv = abs(v);

    if absv < speed1
        regen = 0;
    elseif absv <= speed2
        regen = 0.95*(absv-speed1)/dspeed;
    else
        regen = 0.95;
    end

    if SOC <= 0.8
        SOCfactor = 1;
    elseif SOC < 1
        SOCfactor = 1 - (SOC-0.8)/(1-0.8);
    else
        SOCfactor = 0;
    end

    regen = regen *SOCfactor;

    alpha_PT = a +b*regen;
    alpha_b = b*(1-regen);

end

== matlab function Proj4_FINAL_INDIVIDUAL/Car Body Frame Dynamics/Long Vehicle Dynamics/MATLAB Function ==
  data: F_x input; ax output; M_in input; m input; F_drag input; height input
function ax  = fcn(F_x, M_in, m, F_drag,height)

ax = (F_x - F_drag - m*9.81*sin(atan(height)))/((M_in)+m);

end

== matlab function Proj4_FINAL_INDIVIDUAL/Car Body Frame Dynamics/Proj 3 Calcs/Electric Motor Drive/Battery1/MATLAB Function ==
  data: SOC input; I_bat_min output; I_bat input
function I_bat_min = fcn(SOC, I_bat)
    if SOC <= 0.1
        I_bat_min = 0;
    else
        I_bat_min = I_bat;
    end
end

== matlab function Proj4_FINAL_INDIVIDUAL/Car Body Frame Dynamics/Proj 3 Calcs/Electric Motor Drive/Electric Motor1/MATLAB Function ==
  data: tau_EM input; I_bus output; omega_EM input; eff_EM input; V_bus input
function I_bus = fcn(tau_EM,omega_EM,eff_EM, V_bus)

    Pm = tau_EM*omega_EM;
    sgn_m = sign(Pm);
    Pe = Pm/(eff_EM^sgn_m);
    if V_bus > 1
        I_bus = Pe/V_bus;
    else
        I_bus = 0;
    end
end

== matlab function Proj4_FINAL_INDIVIDUAL/Car Body Frame Dynamics/Proj 3 Calcs/Electric Motor Drive/Inverter1/MATLAB Function ==
  data: V_bat input; V_bus output; I_bat output; eff_I input; I_bus input
function [V_bus, I_bat] = fcn(V_bat, eff_I, I_bus)
    V_bus = V_bat;
    P_bus = V_bus * I_bus;
    sgn_Pbus = P_bus / (abs(P_bus) + 0.001);

    if V_bus > 1
        I_bat = (P_bus / eff_I^sgn_Pbus) / V_bus; 
    else
        I_bat = 0;
    end
end

== matlab function Proj4_FINAL_INDIVIDUAL/Car Body Frame Dynamics/Proj 2 Calcs/MATLAB Function2 ==
  data: vy input; vx input; alpha_f output; delta_f input; axel_distances input; omega input; alpha_r output
function [alpha_f,alpha_r] = slip_angle(vy, vx, delta_f, axel_distances, omega)

    %pulling out lf and lr from defined car parameters
    lf = axel_distances(1);
    lr = axel_distances(2);
    
    epsilon = 0.01*sign(vx);

    %calculating slip angles using all inputs
    alpha_f = delta_f - ((vy + lf * omega)/(vx +epsilon));
    alpha_r = -((vy - lr * omega)/(vx+epsilon));

end

== matlab function Proj4_FINAL_INDIVIDUAL/Car Body Frame Dynamics/Proj 3 Calcs/Brakes/MATLAB Function ==
  data: tau_b output; alpha_b input; N_b_max input; g_b input; mu_b input; omega_w input; tau_w input
function tau_b = fcn(alpha_b, N_b_max, g_b, mu_b,omega_w, tau_w)

tau_b = -mu_b*N_b_max*alpha_b*g_b*sign(omega_w);
end

== matlab function Proj4_FINAL_INDIVIDUAL/Car Body Frame Dynamics/Proj 2 Calcs/MATLAB Function1 ==
  data: Fyf output; Fyr output; alpha_f input; alpha_r input; stiffs input
function [Fyf,Fyr]  = forces(alpha_f, alpha_r, stiffs)

    cf = stiffs(1);
    cr = stiffs(2);

    Fyf = cf* alpha_f;
    Fyr = cr* alpha_r;

end

== matlab function Proj4_FINAL_INDIVIDUAL/Car Body Frame Dynamics/Proj 2 Calcs/MATLAB Function ==
  data: vx input; Fyf input; Fyr input; mass_inert input; axel_distances input; vy_dot output; omega input; omega_dot output
function [vy_dot,omega_dot] = lat_dynamics(vx, Fyf, Fyr, mass_inert, axel_distances, omega)

    lf = axel_distances(1);
    lr = axel_distances(2);
    m = mass_inert(1);
    I = mass_inert(2);

    vy_dot = vx * omega + ((Fyf + Fyr) / m);

    omega_dot = (Fyf * lf - Fyr * lr) / I;

== matlab function Proj4_FINAL_INDIVIDUAL/Driver/MATLAB Function2 ==
  data: X input; Y input; delta_f output; x_center input; y_center input; psi input; v_d output; prev_delta_out output; axel_distances input; v_max input; prev_delta_in input; l input
function [delta_f, v_d, prev_delta_out] = compute_delta_f(X, Y, x_center, y_center,psi, axel_distances, v_max, prev_delta_in,l)
     % Vehicle parameters
    L = axel_distances(1) + axel_distances(2);  % Total wheelbase
    alpha = 300;

    dx = gradient(x_center);
    dy = gradient(y_center);
    ddx = gradient(dx);
    ddy = gradient(dy);

    curvature = abs(dx .* ddy - dy .* ddx) ./ (dx.^2 + dy.^2).^(3/2);
    
    distances = (x_center-X).^2 + (y_center -Y).^2;
    [~, idx] = min(distances);
    kappa = curvature(idx);


    idx2 = min(idx + round(l), length(x_center));
    x_desired = x_center(idx2);
    y_desired = y_center(idx2);

    psi_d = atan2(y_desired - Y, x_desired - X);

    error = psi_d - psi;
    error = atan2(sin(error), cos(error));

    delta_f = atan2(2 * L * sin(error), l);
    max_rate = 0.1;
    delta_f = max(min(delta_f, prev_delta_in + max_rate), prev_delta_in - max_rate);
    prev_delta_out = delta_f;

    v_d = v_max / (1 + alpha * kappa);
    v_d = max(1, min(v_d, v_max));



end

== matlab function Proj4_FINAL_INDIVIDUAL/Driver/MATLAB Function1 ==
  data: X input; height output
function height = fcn(X)

height = 10 * exp((X - 450) / 50) ./ (1 + exp((X - 450) / 50));

end

== matlab function Proj4_FINAL_INDIVIDUAL/Car Body Frame Dynamics/Proj 3 Calcs/ /Drag_force ==
  data: v input; rho input; F_drag output; A input; C_d input; c_1 input; c_0 input
function F_drag = fcn(v, rho, A, C_d, c_1, c_0)

c_2 = 0.5*rho*A*C_d;

F_drag = (v^2)*(c_2) + v*c_1 + c_0;

end
